simulink model "untitled"  (R2016a)
settings: Solver=VariableStepAuto  StartTime=0.0  StopTime=10.0  RelTol=1e-3
libraries: neural x419
(part 1 of 5)
settings Model: Creator=Administrator  LastModifiedBy=Administrator
settings GRTTargetCC: GeneratePreprocessorConditionals=Use local settings

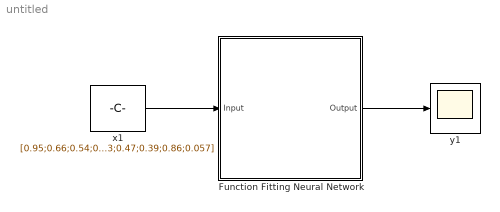
== system untitled ==
  Function Fitting Neural Network : Subsystem
      mask help: Function Fitting Neural Network
      mask Display: e = 0.06;c1 = [120 150 230]/255;c2 = ([120 150 230]+0)/383;c3 = ([120 150 230]+128)/383;patch([0 1 1 0],[0 0 1 1],c1);patch([0 1 1 1-e 1-e 0+e],[0 0 1 1-e 0+e 0+e],c2);patch([0 0 1 1-e 0+e 0+e],[0 1 1 1-e 1-e 0+e],c3);plot([0 1 1 0 0],[0 0 1 1 0]);fprintf('NNET');port_label('input',1,' Input');port_label('output',1,'Output ');
  x1 : Constant  Value=[0.95;0.66;0.54;0.6;0.23;0.82;0.79;0.59;0.44;0.55;0.35;1;0.36;0.97;0.025;0.78;0.44;0.63;0.31;0.92;0.22;0.37;0.31;0.038;0.61;0.84;0.59;0.36;0.14;0.12;0.98;0.54;0.087;0.26;0.21;0.31;0.9;0.52;0.16;0.14;0.064;0.85;0.97;0.93;0.41;0.9;0.48;0.47;0.17;0.083;0.63;0.31;0.47;0.21;0.0014;0.8;0.37;0.015;0.71;0.22;0.69;0.25;0.27;0.13;0.34;0.75;0.89;0.71;0.25;0.45;0.93;0.62;0.26;0.63;0.7;0.4;0.19;0.31;0.69;0.63;0.25;0.043;0.53;0.18;0.52;0.87;0.61;0.27;0.85;0.16;0.26;0.67;0.23;0.83;0.32;0.49;0.76;0.74;0.64;0.25;0.73;0.34;0.3;0.13;0.01;0.92;0.91;0.38;0.7;0.67;0.13;0.2;0.9;0.89;0.38;0.25;0.6;0.63;0.02;0.82;0.52;0.91;0.12;0.95;0.93;0.095;0.42;0.32;0.85;0.95;0.73;0.68;0.64;0.32;0.73;0.16;0.76;0.092;0.97;0.61;0.89;0.19;0.99;0.24;0.22;0.4;0.78;0.84;0.41;0.4;0.77;0.25;0.87;0.68;0.98;0.19;0.22;0.31;0.75;0.37;0.6;0.38;0.55;0.39;0.67;0.015;0.81;0.35;0.72;0.96;0.51;0.67;0.43;0.85;0.65;0.5;0.37;0.69;0.099;0.048;0.87;0.65;0.61;0.42;0.5;0.16;0.093;0.69;0.14;0.53;0.0036;0.43;0.22;0.66;0.5;0.6;0.2;0.14;0.024;0.94;0.7;0.55;0.3;0.043;0.85;0.6;0.019;0.93;0.0098;0.64;0.79;0.53;0.29;0.63;0.43;0.55;0.19;0.74;0.21;0.1;0.9;0.82;0.88;0.088;0.7;0.17;0.83;0.73;0.78;0.76;0.057;0.61;0.9;0.52;0.51;0.26;0.97;0.58;0.97;0.041;0.19;0.52;0.64;0.34;0.65;0.36;0.85;0.54;0.67;0.26;0.12;0.041;0.89;0.75;0.8;0.44;0.075;0.15;0.25;0.079;0.85;0.16;0.62;0.53;0.19;0.76;0.61;0.15;0.45;0.68;0.28;0.62;0.94;0.57;0.69;0.98;0.9;0.65;0.98;0.16;0.51;0.63;0.8;0.42;0.055;0.52;0.13;0.37;0.7;0.13;0.79;0.05;0.82;0.87;0.2;0.61;1;0.042;0.14;0.22;0.58;0.67;0.72;0.5;0.64;0.036;0.19;0.75;0.31;0.75;0.85;0.099;0.6;0.72;0.57;0.24;0.91;0.95;0.52;0.71;0.8;0.2;0.11;0.62;0.022;0.038;0.12;0.82;0.38;0.23;0.37;0.17;0.77;0.33;0.32;0.72;0.58;0.78;0.36;0.18;0.57;0.48;0.42;0.32;0.97;0.26;0.57;0.35;0.31;0.0094;0.67;0.89;0.42;0.86;0.95;0.38;0.2;0.18;0.31;0.85;0.53;0.83;0.11;0.62;0.57;0.26;0.0023;0.29;0.82;0.9;1;0.0084;0.73;0.085;0.63;0.81;0.83;0.57;0.26;0.78;0.17;0.27;0.0049;0.4;0.027;0.85;0.2;0.86;0.056;0.22;0.045;0.75;0.7;0.92;0.91;0.81;1;0.8;0.32;0.025;0.73;0.47;0.39;0.86;0.057]  SampleTime=1
      mask Display: e = 0.06;c1 = [120 230 180]/255;c2 = ([120 230 180]+0)/(256+128);c3 = ([120 230 180]+128)/(256+128);patch([0 1 1 0],[0 0 1 1],c1);patch([0 1 1 1-e 1-e 0+e],[0 0 1 1-e 0+e 0+e],c2);patch([0 0 1 1-e 0+e 0+e],[0 1 1 1-e 1-e 0+e],c3);plot([0 1 1 0 0],[0 0 1 1 0]);disp('Constant');
  y1 : Scope
      mask Display: e = 0.06;c1 = [120 230 180]/255;c2 = ([120 230 180]+0)/(256+128);c3 = ([120 230 180]+128)/(256+128);patch([0 1 1 0],[0 0 1 1],c1);patch([0 1 1 1-e 1-e 0+e],[0 0 1 1-e 0+e 0+e],c2);patch([0 0 1 1-e 0+e 0+e],[0 1 1 1-e 1-e 0+e],c3);plot([0 1 1 0 0],[0 0 1 1 0]);plot([0.15 0.85 0.85 0.15 0.15],[0.5 0.5 0.85 0.85 0.5]);
  wires:
  x1/1 -> Function Fitting Neural Network/1(Input)
  Function Fitting Neural Network/1(Output) -> y1/1

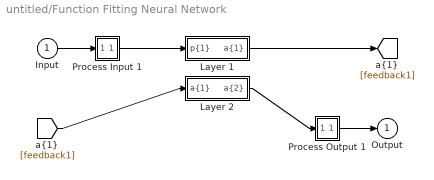
== system untitled/Function Fitting Neural Network ==
  Input : Inport  PortDimensions=405
      mask Display: e = 0.06;c1 = [120 230 180]/255;c2 = ([120 230 180]+0)/(256+128);c3 = ([120 230 180]+128)/(256+128);patch([0 1 1 0],[0 0 1 1],c1);patch([0 1 1 1-e 1-e 0+e],[0 0 1 1-e 0+e 0+e],c2);patch([0 0 1 1-e 0+e 0+e],[0 1 1 1-e 1-e 0+e],c3);plot([0 1 1 0 0],[0 0 1 1 0]);
  Layer 1 : Subsystem
      mask Display: e = 0.06;c1 = [120 150 230]/255;c2 = ([120 150 230]+0)/383;c3 = ([120 150 230]+128)/383;patch([0 1 1 0],[0 0 1 1],c1);patch([0 1 1 1-e 1-e 0+e],[0 0 1 1-e 0+e 0+e],c2);patch([0 0 1 1-e 0+e 0+e],[0 1 1 1-e 1-e 0+e],c3);plot([0 1 1 0 0],[0 0 1 1 0]);
  Layer 2 : Subsystem
      mask Display: e = 0.06;c1 = [120 150 230]/255;c2 = ([120 150 230]+0)/383;c3 = ([120 150 230]+128)/383;patch([0 1 1 0],[0 0 1 1],c1);patch([0 1 1 1-e 1-e 0+e],[0 0 1 1-e 0+e 0+e],c2);patch([0 0 1 1-e 0+e 0+e],[0 1 1 1-e 1-e 0+e],c3);plot([0 1 1 0 0],[0 0 1 1 0]);
  Process Input 1 : Subsystem
      mask Display: e = 0.06;c1 = [120 150 230]/255;c2 = ([120 150 230]+0)/383;c3 = ([120 150 230]+128)/383;patch([0 1 1 0],[0 0 1 1],c1);patch([0 1 1 1-e 1-e 0+e],[0 0 1 1-e 0+e 0+e],c2);patch([0 0 1 1-e 0+e 0+e],[0 1 1 1-e 1-e 0+e],c3);plot([0 1 1 0 0],[0 0 1 1 0]);
  Process Output 1 : Subsystem
      mask Display: e = 0.06;c1 = [120 150 230]/255;c2 = ([120 150 230]+0)/383;c3 = ([120 150 230]+128)/383;patch([0 1 1 0],[0 0 1 1],c1);patch([0 1 1 1-e 1-e 0+e],[0 0 1 1-e 0+e 0+e],c2);patch([0 0 1 1-e 0+e 0+e],[0 1 1 1-e 1-e 0+e],c3);plot([0 1 1 0 0],[0 0 1 1 0]);
  Output : Outport  InitialOutput=[0;0;0;0;0;0;0;0;0;0;0;0;0;0;0;0;0;0;0;0;0;0;0;0;0;0;0;0;0;0;0;0;0;0;0;0;0;0;0;0;0;0;0;0;0;0;0;0;0;0;0;0;0;0;0;0;0;0;0;0;0;0;0;0;0;0;0;0;0;0;0;0;0;0;0;0;0;0;0;0;0;0;0;0;0;0;0;0;0;0;0;0;0;0;0;0;0;0;0;0;0;0;0;0;0;0;0;0;0;0;0;0;0;0;0;0;0;0;0;0;0;0;0;0;0;0;0;0;0;0;0;0;0;0;0;0;0;0;0;0;0;0;0;0;0;0;0;0;0;0;0;0;0;0;0;0;0;0;0;0;0;0;0;0;0;0;0;0;0;0;0;0;0;0;0;0;0;0;0;0;0;0;0;0;0;0;0;0;0;0;0;0;0;0;0;0;0;0;0;0;0;0;0;0;0;0;0;0;0;0;0;0;0;0;0;0;0;0;0;0;0;0;0;0;0;0;0;0;0;0;0;0;0;0;0;0;0;0;0;0;0;0;0;0;0;0;0;0;0;0;0;0;0;0;0;0;0;0;0;0;0;0;0;0;0;0;0;0;0;0;0;0;0;0;0;0;0;0;0;0;0;0;0;0;0;0;0;0;0;0;0;0;0;0;0;0;0;0;0;0;0;0;0;0;0;0;0;0;0;0;0;0;0;0;0;0;0;0;0;0;0;0;0;0;0;0;0;0;0;0;0;0;0;0;0;0;0;0;0;0;0;0;0;0;0;0;0;0;0;0;0;0;0;0;0;0;0;0;0;0;0;0;0;0;0;0;0;0;0;0;0;0;0;0;0;0;0;0;0;0;0;0;0;0;0;0;0;0;0;0;0;0;0;0;0;0;0;0;0;0;0;0;0;0;0]
      mask Display: e = 0.06;c1 = [120 230 180]/255;c2 = ([120 230 180]+0)/(256+128);c3 = ([120 230 180]+128)/(256+128);patch([0 1 1 0],[0 0 1 1],c1);patch([0 1 1 1-e 1-e 0+e],[0 0 1 1-e 0+e 0+e],c2);patch([0 0 1 1-e 0+e 0+e],[0 1 1 1-e 1-e 0+e],c3);plot([0 1 1 0 0],[0 0 1 1 0]);
  wires:
  Input/1 -> Process Input 1/1(x)
  Process Output 1/1(y) -> Output/1
  Process Input 1/1(p) -> Layer 1/1("p{1}")
  Layer 1/1("a{1}") -> [feedback1]
  [feedback1] -> Layer 2/1("a{1} ")
  Layer 2/1("a{2}") -> Process Output 1/1(a)

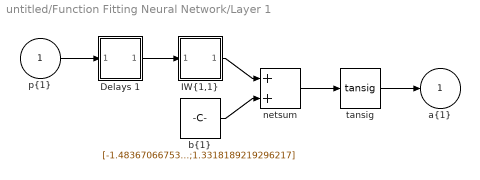
== system untitled/Function Fitting Neural Network/Layer 1 ==
  "p{1}" : Inport  PortDimensions=405
      mask Display: e = 0.06;c1 = [120 230 180]/255;c2 = ([120 230 180]+0)/(256+128);c3 = ([120 230 180]+128)/(256+128);patch([0 1 1 0],[0 0 1 1],c1);patch([0 1 1 1-e 1-e 0+e],[0 0 1 1-e 0+e 0+e],c2);patch([0 0 1 1-e 0+e 0+e],[0 1 1 1-e 1-e 0+e],c3);plot([0 1 1 0 0],[0 0 1 1 0]);
  Delays 1 : Subsystem
      mask Display: e = 0.06;c1 = [120 150 230]/255;c2 = ([120 150 230]+0)/383;c3 = ([120 150 230]+128)/383;patch([0 1 1 0],[0 0 1 1],c1);patch([0 1 1 1-e 1-e 0+e],[0 0 1 1-e 0+e 0+e],c2);patch([0 0 1 1-e 0+e 0+e],[0 1 1 1-e 1-e 0+e],c3);plot([0 1 1 0 0],[0 0 1 1 0]);disp('0');
  "IW{1,1}" : Subsystem
      mask Display: e = 0.06;c1 = [120 150 230]/255;c2 = ([120 150 230]+0)/383;c3 = ([120 150 230]+128)/383;patch([0 1 1 0],[0 0 1 1],c1);patch([0 1 1 1-e 1-e 0+e],[0 0 1 1-e 0+e 0+e],c2);patch([0 0 1 1-e 0+e 0+e],[0 1 1 1-e 1-e 0+e],c3);plot([0 1 1 0 0],[0 0 1 1 0]);disp('W');
  "b{1}" : Constant  Value=[-1.4836706675333449;1.1047984464897049;0.89622700888897611;0.1552630754069747;-0.11692081968564359;-0.69997059175300758;-0.31372259978451555;0.40436973743077254;0.88872224330216254;1.3318189219296217]
      mask Display: e = 0.06;c1 = [120 150 230]/255;c2 = ([120 150 230]+0)/383;c3 = ([120 150 230]+128)/383;patch([0 1 1 0],[0 0 1 1],c1);patch([0 1 1 1-e 1-e 0+e],[0 0 1 1-e 0+e 0+e],c2);patch([0 0 1 1-e 0+e 0+e],[0 1 1 1-e 1-e 0+e],c3);plot([0 1 1 0 0],[0 0 1 1 0]);disp('b');
  netsum : Sum  Inputs=2  SaturateOnIntegerOverflow=on  InputSameDT=on  OutDataTypeStr=Inherit: Same as first input
      mask Display: e = 0.06;c1 = [120 150 230]/255;c2 = ([120 150 230]+0)/383;c3 = ([120 150 230]+128)/383;patch([0 1 1 0],[0 0 1 1],c1);patch([0 1 1 1-e 1-e 0+e],[0 0 1 1-e 0+e 0+e],c2);patch([0 0 1 1-e 0+e 0+e],[0 1 1 1-e 1-e 0+e],c3);plot([0 1 1 0 0],[0 0 1 1 0]);disp('+');
  tansig : neural/Transfer Functions/tansig
  "a{1}" : Outport  InitialOutput=[0;0;0;0;0;0;0;0;0;0]
      mask Display: e = 0.06;c1 = [120 230 180]/255;c2 = ([120 230 180]+0)/(256+128);c3 = ([120 230 180]+128)/(256+128);patch([0 1 1 0],[0 0 1 1],c1);patch([0 1 1 1-e 1-e 0+e],[0 0 1 1-e 0+e 0+e],c2);patch([0 0 1 1-e 0+e 0+e],[0 1 1 1-e 1-e 0+e],c3);plot([0 1 1 0 0],[0 0 1 1 0]);
  wires:
  "p{1}"/1 -> Delays 1/1("p{1}")
  Delays 1/1("pd{1,1}") -> "IW{1,1}"/1("pd{1,1}")
  "IW{1,1}"/1("iz{1,1}") -> netsum/1
  "b{1}"/1 -> netsum/2
  netsum/1 -> tansig/1
  tansig/1 -> "a{1}"/1

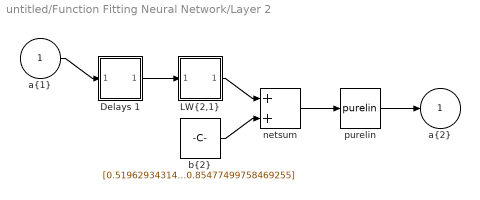
== system untitled/Function Fitting Neural Network/Layer 2 ==
  "a{1} " : Inport  PortDimensions=10
      mask Display: e = 0.06;c1 = [120 230 180]/255;c2 = ([120 230 180]+0)/(256+128);c3 = ([120 230 180]+128)/(256+128);patch([0 1 1 0],[0 0 1 1],c1);patch([0 1 1 1-e 1-e 0+e],[0 0 1 1-e 0+e 0+e],c2);patch([0 0 1 1-e 0+e 0+e],[0 1 1 1-e 1-e 0+e],c3);plot([0 1 1 0 0],[0 0 1 1 0]);
  Delays 1 : Subsystem
      mask Display: e = 0.06;c1 = [120 150 230]/255;c2 = ([120 150 230]+0)/383;c3 = ([120 150 230]+128)/383;patch([0 1 1 0],[0 0 1 1],c1);patch([0 1 1 1-e 1-e 0+e],[0 0 1 1-e 0+e 0+e],c2);patch([0 0 1 1-e 0+e 0+e],[0 1 1 1-e 1-e 0+e],c3);plot([0 1 1 0 0],[0 0 1 1 0]);disp('0');
  "LW{2,1}" : Subsystem
      mask Display: e = 0.06;c1 = [120 150 230]/255;c2 = ([120 150 230]+0)/383;c3 = ([120 150 230]+128)/383;patch([0 1 1 0],[0 0 1 1],c1);patch([0 1 1 1-e 1-e 0+e],[0 0 1 1-e 0+e 0+e],c2);patch([0 0 1 1-e 0+e 0+e],[0 1 1 1-e 1-e 0+e],c3);plot([0 1 1 0 0],[0 0 1 1 0]);disp('W');
  "b{2}" : Constant  Value=[0.51962934314456621;0.62722310510799217;0.0039625582046517588;0.44530598532349275;0.23909666427167295;-0.11512102998395637;-0.18368252804419391;0.32340506918540196;0.22170992472783632;-0.30750296856810738;0.36563940725531047;0.40252199282885848;0.31399071882226176;0.24664882700903951;0.10127502899071568;0.56482493071667961;0.10871603996857498;0.64555958501338695;-0.10839199260549295;0.0063244715717595823;-0.78634602645471752;0.42763027139322246;0.36641870556114342;0.27567465914204453;0.090872018229214813;0.090524849711426256;-0.22796381050837947;0.23075660800946271;0.42633613365994033;-0.048423185921140949;0.12913169657994977;0.41654136269123698;0.3589684745964612;0.20690076108044331;-0.18289258350496218;-0.81558824843377131;-0.6365116202342066;0.32864625819226068;-0.022199334341076946;0.13109549080111804;-0.43166338327279269;0.49877671371532795;0.033048073167747896;-0.45083087457285143;0.29293382878572161;0.057353820948484208;0.65924302003961288;0.55520685124121338;0.48248142971274011;0.27698734640101025;0.3417941962793335;0.12921532031479316;0.081712615273866751;0.20275573058319929;0.34677400328843416;0.55005328557584499;-0.012334043990333943;-0.38247925036535368;-0.49064590813227538;-0.15439573104858154;0.17174272840030774;-0.2511309730722967;-0.19180330291534842;0.083763544446833621;-0.07020123484685703;-0.60882101630607643;-0.045721539251927248;-0.45195477431436193;0.431656301454731;-0.0051718042464756336;0.40238656350072322;0.081458486534659563;-0.22796485308413603;-0.25581762638741257;-0.039398598701752996;-0.085612981033651725;-0.34314089976655787;-0.49843651053771115;0.54521383671853296;-0.44844972841403175;-0.26082353346135972;-0.043971882992698538;0.38310651442848959;-0.18182237518452857;0.8209131208285898;0.14394286713996646;-0.13092896227242465;0.78663376920457373;-0.04647565808773902;0.81865633551518613;0.46290774202068413;0.49673151255871134;-0.1655423169847027;-0.056073093845701714;0.63536195260871187;0.13813947760869516;0.76840245586626565;0.18794280437895977;0.51655583332025645;0.12970158334624471;0.28447181110750364;0.6179031114131317;0.27669918194144771;0.41875242269758461;0.12629212375037574;-0.17700474915586167;-0.19954002126125658;0.30502318032852271;0.026528614951103924;-0.18201626846527177;0.10956687661115558;0.38190973069058887;-0.3283079520810267;0.56825640661178323;-0.10853033001431761;-0.2411644179998749;-0.066107198541484363;-0.025534530870895467;-0.3940115167571081;-0.5264490777387868;0.95445238123324816;0.79919563645720015;-0.4290825099469876;0.51739719168116882;-0.46360577417934795;1.0592444909773437;0.12513078732201494;-0.61031948395019342;0.061506205968693245;0.13045913084973643;-0.47270007969866201;0.44218223381196209;0.45615687788062398;-0.49970424890224102;0.92557958050815192;0.35043580769689109;-0.33443948587870603;0.00016426272557737431;-0.19722349632121378;0.030993564889854441;-0.22169681406076003;0.1826373317900386;-0.12774423591991324;0.34155769032447619;0.52379485995905783;0.20845274323966106;0.2552366738685713;-0.15529540819003285;-0.0091727910214912667;-0.15983024712490465;0.66110078155355856;0.52530681016846559;0.25980766599382921;0.62916754327010371;0.70071578215292341;-0.37548149786719554;0.31153877625486381;0.82416272151710812;-0.28783600167484502;0.24873588356389056;0.79790769522420291;0.036957234761960722;-0.65391130638544981;0.23927121833997295;0.28173722764832965;-0.31259053834318318;0.084116983240382526;-0.44059316637300039;-0.3863849856621755;-0.16982913856810194;-0.93120833709291084;0.048057270508828472;0.64414325230631486;0.22502272389569047;-0.21255717029782562;0.76932627040393531;0.49662801172448828;-0.33805986527216053;0.015555228342185052;-0.32913413883039233;0.23220507928921397;0.31589360806868605;-0.51329559787326462;0.30245110772626793;0.25841279086892971;-0.037852577738636095;-0.39038441511393202;-0.68491982900800397;0.60950074562076972;-0.74430955489317951;0.12498068514470491;-0.48148505198279906;0.10074590190399084;0.20171908172067216;-0.79511283130895993 ...(+4290 chars)]
      mask Display: e = 0.06;c1 = [120 150 230]/255;c2 = ([120 150 230]+0)/383;c3 = ([120 150 230]+128)/383;patch([0 1 1 0],[0 0 1 1],c1);patch([0 1 1 1-e 1-e 0+e],[0 0 1 1-e 0+e 0+e],c2);patch([0 0 1 1-e 0+e 0+e],[0 1 1 1-e 1-e 0+e],c3);plot([0 1 1 0 0],[0 0 1 1 0]);disp('b');
  netsum : Sum  Inputs=2  SaturateOnIntegerOverflow=on  InputSameDT=on  OutDataTypeStr=Inherit: Same as first input
      mask Display: e = 0.06;c1 = [120 150 230]/255;c2 = ([120 150 230]+0)/383;c3 = ([120 150 230]+128)/383;patch([0 1 1 0],[0 0 1 1],c1);patch([0 1 1 1-e 1-e 0+e],[0 0 1 1-e 0+e 0+e],c2);patch([0 0 1 1-e 0+e 0+e],[0 1 1 1-e 1-e 0+e],c3);plot([0 1 1 0 0],[0 0 1 1 0]);disp('+');
  purelin : neural/Transfer Functions/purelin
  "a{2}" : Outport  InitialOutput=[0;0;0;0;0;0;0;0;0;0;0;0;0;0;0;0;0;0;0;0;0;0;0;0;0;0;0;0;0;0;0;0;0;0;0;0;0;0;0;0;0;0;0;0;0;0;0;0;0;0;0;0;0;0;0;0;0;0;0;0;0;0;0;0;0;0;0;0;0;0;0;0;0;0;0;0;0;0;0;0;0;0;0;0;0;0;0;0;0;0;0;0;0;0;0;0;0;0;0;0;0;0;0;0;0;0;0;0;0;0;0;0;0;0;0;0;0;0;0;0;0;0;0;0;0;0;0;0;0;0;0;0;0;0;0;0;0;0;0;0;0;0;0;0;0;0;0;0;0;0;0;0;0;0;0;0;0;0;0;0;0;0;0;0;0;0;0;0;0;0;0;0;0;0;0;0;0;0;0;0;0;0;0;0;0;0;0;0;0;0;0;0;0;0;0;0;0;0;0;0;0;0;0;0;0;0;0;0;0;0;0;0;0;0;0;0;0;0;0;0;0;0;0;0;0;0;0;0;0;0;0;0;0;0;0;0;0;0;0;0;0;0;0;0;0;0;0;0;0;0;0;0;0;0;0;0;0;0;0;0;0;0;0;0;0;0;0;0;0;0;0;0;0;0;0;0;0;0;0;0;0;0;0;0;0;0;0;0;0;0;0;0;0;0;0;0;0;0;0;0;0;0;0;0;0;0;0;0;0;0;0;0;0;0;0;0;0;0;0;0;0;0;0;0;0;0;0;0;0;0;0;0;0;0;0;0;0;0;0;0;0;0;0;0;0;0;0;0;0;0;0;0;0;0;0;0;0;0;0;0;0;0;0;0;0;0;0;0;0;0;0;0;0;0;0;0;0;0;0;0;0;0;0;0;0;0;0;0;0;0;0;0;0;0;0;0;0;0;0;0;0;0;0;0;0]
      mask Display: e = 0.06;c1 = [120 230 180]/255;c2 = ([120 230 180]+0)/(256+128);c3 = ([120 230 180]+128)/(256+128);patch([0 1 1 0],[0 0 1 1],c1);patch([0 1 1 1-e 1-e 0+e],[0 0 1 1-e 0+e 0+e],c2);patch([0 0 1 1-e 0+e 0+e],[0 1 1 1-e 1-e 0+e],c3);plot([0 1 1 0 0],[0 0 1 1 0]);
  wires:
  "a{1} "/1 -> Delays 1/1("p{2}")
  Delays 1/1("pd{2,1}") -> "LW{2,1}"/1("ad{2,1}")
  "LW{2,1}"/1("lz{2,1}") -> netsum/1
  "b{2}"/1 -> netsum/2
  netsum/1 -> purelin/1
  purelin/1 -> "a{2}"/1

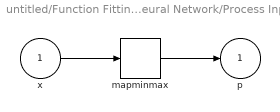
== system untitled/Function Fitting Neural Network/Process Input 1 ==
  x : Inport  PortDimensions=405
      mask Display: e = 0.06;c1 = [120 230 180]/255;c2 = ([120 230 180]+0)/(256+128);c3 = ([120 230 180]+128)/(256+128);patch([0 1 1 0],[0 0 1 1],c1);patch([0 1 1 1-e 1-e 0+e],[0 0 1 1-e 0+e 0+e],c2);patch([0 0 1 1-e 0+e 0+e],[0 1 1 1-e 1-e 0+e],c3);plot([0 1 1 0 0],[0 0 1 1 0]);
  mapminmax : neural/Processing Functions/mapminmax  xmin=[-85;-85;-85;-85;-85;-86;-80;-84;-84;-80;-80;-84;-85;-84;0;-84;-80;0;0;-10;-34;0;0;0;0;-47;0;0;0;0;0;0;0;0;0;0;0;0;0;0;0;0;0;0;-37;-84;-74;-81;-81;-80;-80;0;-63;-41;0;0;0;0;0;-84;-84;0;0;0;0;0;0;0;-41;-41;0;-41;0;-9;0;-10;0;-47;0;-46;0;-1;-34;-20;-1;-39;-1;-58;-51;-8;-46;-77;-79;-47;-58;-58;-58;-57;-58;-57;-58;-57;-38;-58;-58;-58;-58;-58;-58;-58;-57;-58;-58;-58;-58;-56;-58;-58;-58;-53;-83;-58;-58;-37;-64;-70;-58;-50;-50;-53;-56;-45;-40;-52;-58;-58;-34;-41;-41;-64;-58;-58;-56;-43;-57;-59;-57;-55;-58;-58;-58;-57;-58;-58;-58;-58;-58;-46;-38;-43;-58;-58;-73;-75;-81;-89;-80;-89;-86;-71;-86;-76;-78;-78;-86;-81;-78;-77;-73;-86;-79;-82;-74;-82;-69;-87;-88;-85;-54;-64;-68;-80;-86;-87;-69;-66;-45;-87;-84;-65;-63;-67;-61;-88;-81;-80;-83;-80;-81;-78;-58;-72;-86;-85;-81;-83;-87;-79;-85;-89;-86;-77;-76;-85;-77;-74;-81;-74;-78;-78;-79;-77;-82;-85;-80;-85;-75;-80;-84;-81;-81;-80;-81;-80;-79;-80;-75;-81;-77;-78;-77;-76;-77;-75;-82;-76;-82;-79;-77;-86;-82;-77;-78;-81;-77;-77;-79;-80;-80;-79;-82;-79;-78;-76;-75;-78;-75;-82;-82;-81;-81;-84;-79;-77;-76;-80;-81;-77;-82;-80;-78;-82;-77;-80;-85;-79;-80;-80;-82;-78;-77;-76;-77;-82;-81;-82;-84;-85;-79;-77;-80;-82;-81;-78;-86;-86;-80;-80;-82;-82;-80;-82;-80;-78;0;0;0;0;0;0;0;-1;0;0;0;-85;-85;-80;-80;-85;-84;0;0;0;0;0;0;-1;0;0;0;0;0;0;0;0;0;0;0;0;0;0;0;0;0;0;0;0;0;0;0;0;0;0;0;0;0;0;0;0;0;0;0;0;0;0;0;0;0;0;0;0;0;0;0;0;0;0;0;0;0;0;0;0;0]  xmax=[317;317;317;317;318;318;318;318;318;319;322;322;322;327;334;337;327;301;291;290;288;291;292;292;294;296;297;298;298;299;297;298;297;298;297;298;298;297;297;295;294;291;287;285;284;280;275;266;263;267;274;282;290;294;298;300;305;309;308;309;310;307;304;302;296;293;292;291;292;293;292;292;292;292;292;292;292;291;292;293;293;291;291;289;291;290;290;283;278;275;272;273;272;274;277;280;279;281;282;281;282;282;283;282;282;281;281;282;282;283;281;283;282;284;284;284;284;283;284;284;284;284;284;285;286;285;284;285;285;285;284;285;285;285;284;284;285;285;286;286;285;284;285;285;284;286;284;285;284;285;285;285;284;285;284;286;285;284;285;283;285;284;285;286;286;287;286;284;283;279;281;280;280;277;279;282;283;282;281;283;286;286;287;287;286;287;286;285;285;285;284;283;283;283;284;284;284;284;284;283;284;285;284;283;283;283;283;285;284;284;283;285;283;284;283;283;283;283;284;284;283;282;282;282;283;283;283;283;282;282;282;283;282;281;281;281;281;281;280;281;280;280;279;281;282;283;284;282;283;283;282;283;282;283;283;283;282;283;282;282;282;282;283;282;282;282;283;283;282;283;282;283;282;283;282;283;282;282;281;282;281;281;282;283;282;283;283;283;283;283;281;283;283;282;282;282;282;282;282;283;283;283;282;282;283;283;282;282;282;282;282;282;283;283;282;281;282;282;282;281;281;282;281;282;288;291;294;299;302;302;306;307;305;306;307;315;321;322;320;317;314;308;303;300;298;296;295;294;295;294;293;296;295;296;296;296;298;298;299;299;298;299;299;300;300;299;299;299;299;299;300;300;299;299;299;299;299;299;300;299;298;298;298;298;297;298;298;298;298;299;298;299;299;298;299;299;299;297;298;298;299;297;298;298;298]  ymin=-1  ymax=1
  p : Outport  PortDimensions=405
      mask Display: e = 0.06;c1 = [120 230 180]/255;c2 = ([120 230 180]+0)/(256+128);c3 = ([120 230 180]+128)/(256+128);patch([0 1 1 0],[0 0 1 1],c1);patch([0 1 1 1-e 1-e 0+e],[0 0 1 1-e 0+e 0+e],c2);patch([0 0 1 1-e 0+e 0+e],[0 1 1 1-e 1-e 0+e],c3);plot([0 1 1 0 0],[0 0 1 1 0]);
  wires:
  x/1 -> mapminmax/1
  mapminmax/1 -> p/1

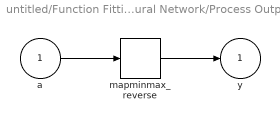
== system untitled/Function Fitting Neural Network/Process Output 1 ==
  a : Inport  PortDimensions=405
      mask Display: e = 0.06;c1 = [120 230 180]/255;c2 = ([120 230 180]+0)/(256+128);c3 = ([120 230 180]+128)/(256+128);patch([0 1 1 0],[0 0 1 1],c1);patch([0 1 1 1-e 1-e 0+e],[0 0 1 1-e 0+e 0+e],c2);patch([0 0 1 1-e 0+e 0+e],[0 1 1 1-e 1-e 0+e],c3);plot([0 1 1 0 0],[0 0 1 1 0]);
  mapminmax_reverse : neural/Processing Functions/mapminmax_reverse  xmin=[-85;-85;-85;-85;-85;-86;-80;-84;-84;-80;-80;-84;-85;-84;0;-84;-80;0;0;-10;-34;0;0;0;0;-47;0;0;0;0;0;0;0;0;0;0;0;0;0;0;0;0;0;0;-37;-84;-74;-81;-81;-80;-80;0;-63;-41;0;0;0;0;0;-84;-84;0;0;0;0;0;0;0;-41;-41;0;-41;0;-9;0;-10;0;-47;0;-46;0;-1;-34;-20;-1;-39;-1;-58;-51;-8;-46;-77;-79;-47;-58;-58;-58;-57;-58;-57;-58;-57;-38;-58;-58;-58;-58;-58;-58;-58;-57;-58;-58;-58;-58;-56;-58;-58;-58;-53;-83;-58;-58;-37;-64;-70;-58;-50;-50;-53;-56;-45;-40;-52;-58;-58;-34;-41;-41;-64;-58;-58;-56;-43;-57;-59;-57;-55;-58;-58;-58;-57;-58;-58;-58;-58;-58;-46;-38;-43;-58;-58;-73;-75;-81;-89;-80;-89;-86;-71;-86;-76;-78;-78;-86;-81;-78;-77;-73;-86;-79;-82;-74;-82;-69;-87;-88;-85;-54;-64;-68;-80;-86;-87;-69;-66;-45;-87;-84;-65;-63;-67;-61;-88;-81;-80;-83;-80;-81;-78;-58;-72;-86;-85;-81;-83;-87;-79;-85;-89;-86;-77;-76;-85;-77;-74;-81;-74;-78;-78;-79;-77;-82;-85;-80;-85;-75;-80;-84;-81;-81;-80;-81;-80;-79;-80;-75;-81;-77;-78;-77;-76;-77;-75;-82;-76;-82;-79;-77;-86;-82;-77;-78;-81;-77;-77;-79;-80;-80;-79;-82;-79;-78;-76;-75;-78;-75;-82;-82;-81;-81;-84;-79;-77;-76;-80;-81;-77;-82;-80;-78;-82;-77;-80;-85;-79;-80;-80;-82;-78;-77;-76;-77;-82;-81;-82;-84;-85;-79;-77;-80;-82;-81;-78;-86;-86;-80;-80;-82;-82;-80;-82;-80;-78;0;0;0;0;0;0;0;-1;0;0;0;-85;-85;-80;-80;-85;-84;0;0;0;0;0;0;-1;0;0;0;0;0;0;0;0;0;0;0;0;0;0;0;0;0;0;0;0;0;0;0;0;0;0;0;0;0;0;0;0;0;0;0;0;0;0;0;0;0;0;0;0;0;0;0;0;0;0;0;0;0;0;0;0;0]  xmax=[317;317;317;317;318;318;318;318;318;319;322;322;322;327;334;337;327;301;291;290;288;291;292;292;294;296;297;298;298;299;297;298;297;298;297;298;298;297;297;295;294;291;287;285;284;280;275;266;263;267;274;282;290;294;298;300;305;309;308;309;310;307;304;302;296;293;292;291;292;293;292;292;292;292;292;292;292;291;292;293;293;291;291;289;291;290;290;283;278;275;272;273;272;274;277;280;279;281;282;281;282;282;283;282;282;281;281;282;282;283;281;283;282;284;284;284;284;283;284;284;284;284;284;285;286;285;284;285;285;285;284;285;285;285;284;284;285;285;286;286;285;284;285;285;284;286;284;285;284;285;285;285;284;285;284;286;285;284;285;283;285;284;285;286;286;287;286;284;283;279;281;280;280;277;279;282;283;282;281;283;286;286;287;287;286;287;286;285;285;285;284;283;283;283;284;284;284;284;284;283;284;285;284;283;283;283;283;285;284;284;283;285;283;284;283;283;283;283;284;284;283;282;282;282;283;283;283;283;282;282;282;283;282;281;281;281;281;281;280;281;280;280;279;281;282;283;284;282;283;283;282;283;282;283;283;283;282;283;282;282;282;282;283;282;282;282;283;283;282;283;282;283;282;283;282;283;282;282;281;282;281;281;282;283;282;283;283;283;283;283;281;283;283;282;282;282;282;282;282;283;283;283;282;282;283;283;282;282;282;282;282;282;283;283;282;281;282;282;282;281;281;282;281;282;288;291;294;299;302;302;306;307;305;306;307;315;321;322;320;317;314;308;303;300;298;296;295;294;295;294;293;296;295;296;296;296;298;298;299;299;298;299;299;300;300;299;299;299;299;299;300;300;299;299;299;299;299;299;300;299;298;298;298;298;297;298;298;298;298;299;298;299;299;298;299;299;299;297;298;298;299;297;298;298;298]  ymin=-1  ymax=1
  y : Outport  PortDimensions=405
      mask Display: e = 0.06;c1 = [120 230 180]/255;c2 = ([120 230 180]+0)/(256+128);c3 = ([120 230 180]+128)/(256+128);patch([0 1 1 0],[0 0 1 1],c1);patch([0 1 1 1-e 1-e 0+e],[0 0 1 1-e 0+e 0+e],c2);patch([0 0 1 1-e 0+e 0+e],[0 1 1 1-e 1-e 0+e],c3);plot([0 1 1 0 0],[0 0 1 1 0]);
  wires:
  a/1 -> mapminmax_reverse/1
  mapminmax_reverse/1 -> y/1

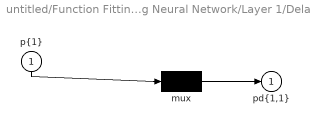
== system untitled/Function Fitting Neural Network/Layer 1/Delays 1 ==
  "p{1}" : Inport  PortDimensions=405
      mask Display: e = 0.06;c1 = [120 230 180]/255;c2 = ([120 230 180]+0)/(256+128);c3 = ([120 230 180]+128)/(256+128);patch([0 1 1 0],[0 0 1 1],c1);patch([0 1 1 1-e 1-e 0+e],[0 0 1 1-e 0+e 0+e],c2);patch([0 0 1 1-e 0+e 0+e],[0 1 1 1-e 1-e 0+e],c3);plot([0 1 1 0 0],[0 0 1 1 0]);
  mux : Mux  Inputs=1
      mask Display: e = 0.06;c1 = [120 150 230]/255;c2 = ([120 150 230]+0)/383;c3 = ([120 150 230]+128)/383;patch([0 1 1 0],[0 0 1 1],c1);patch([0 1 1 1-e 1-e 0+e],[0 0 1 1-e 0+e 0+e],c2);patch([0 0 1 1-e 0+e 0+e],[0 1 1 1-e 1-e 0+e],c3);plot([0 1 1 0 0],[0 0 1 1 0]);disp('Mux')
  "pd{1,1}" : Outport
      mask Display: e = 0.06;c1 = [120 230 180]/255;c2 = ([120 230 180]+0)/(256+128);c3 = ([120 230 180]+128)/(256+128);patch([0 1 1 0],[0 0 1 1],c1);patch([0 1 1 1-e 1-e 0+e],[0 0 1 1-e 0+e 0+e],c2);patch([0 0 1 1-e 0+e 0+e],[0 1 1 1-e 1-e 0+e],c3);plot([0 1 1 0 0],[0 0 1 1 0]);
  wires:
  "p{1}"/1 -> mux/1
  mux/1 -> "pd{1,1}"/1
